simulink model "Model1_1"  (R2015a)
settings: Solver=ode45  StartTime=0.0  StopTime=10.0  RelTol=1e-3
settings Model: Creator=qiji  LastModifiedBy=qiji
settings DebuggingCC: UnderspecifiedInitializationDetection=Classic  MergeDetectMultiDrivingBlocksExec=none  SolverPrmCheckMsg=warning

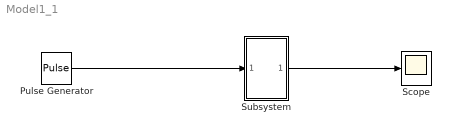
== system Model1_1 ==
  Pulse Generator : DiscretePulseGenerator  Period=5
  Scope : Scope
  Subsystem : Subsystem
  wires:
  Pulse Generator/1 -> Subsystem/1(In1)
  Subsystem/1(Out) -> Scope/1

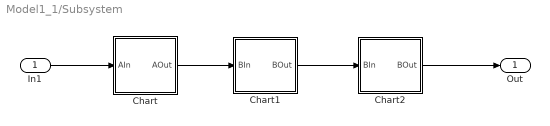
== system Model1_1/Subsystem ==
  In1 : Inport
  Chart : Stateflow chart  TreatAsAtomicUnit=on
  Chart1 : Stateflow chart  TreatAsAtomicUnit=on
  Chart2 : Stateflow chart  TreatAsAtomicUnit=on
  Out : Outport
  wires:
  Chart2/1(BOut) -> Out/1
  Chart/1(AOut) -> Chart1/1(BIn)
  In1/1 -> Chart/1(AIn)
  Chart1/1(BOut) -> Chart2/1(BIn)

== stateflow chart Model1_1/Subsystem/Chart ==
  state A
    en:
    AOut = 0;
  state B
    en:
    AOut = 1;
  A -> B : [AIn == 1]
  (default) -> A
  B -> A : [AIn==1]
  data: AIn input double; AOut output double

== stateflow chart Model1_1/Subsystem/Chart1 ==
  state A
    du:
    BOut = BIn
  (default) -> A
  data: BIn input double; BOut output double

== stateflow chart Model1_1/Subsystem/Chart2 ==
  state A
    du:
    BOut = BIn
  (default) -> A
  data: BIn input double; BOut output double
